simulink model "ex2_4"  (Simulink 7.8)
settings: Solver=ode45  StartTime=0.0  StopTime=1000.0  MaxStep=1  MinStep=1e-3  RelTol=1e-3
libraries: simulink x2
settings Model: Creator=Luke  LastModifiedBy=Luke

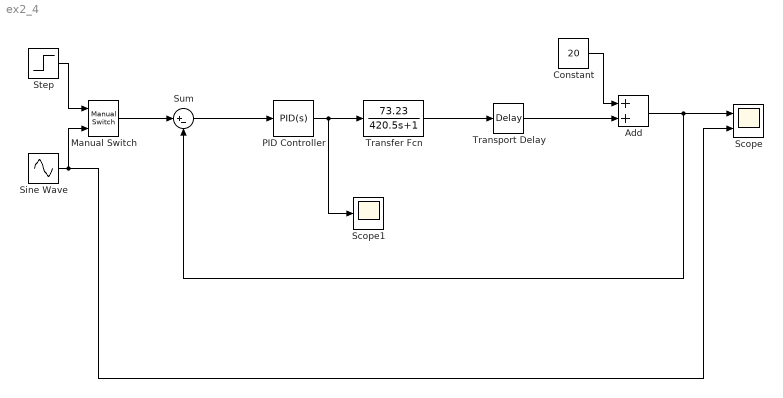
== system ex2_4 ==
  Add : Sum
  Constant : Constant  Value=20
  Manual Switch : simulink/Signal Routing/Manual Switch  sw=1  action=0  varsize=off
  PID Controller : simulink/Continuous/PID Controller  Controller=PID  TimeDomain=Continuous-time  SampleTime=1  IntegratorMethod=Forward Euler  FilterMethod=Forward Euler  Form=Parallel  P=0.6*0.2  I=(1.2*0.2)/110  D=(3*0.2*110)/40  N=15  InitialConditionSource=internal  InitialConditionForIntegrator=0  InitialConditionForFilter=0  ExternalReset=none  LimitOutput=off  UpperSaturationLimit=inf  LowerSaturationLimit=-inf  LinearizeAsGain=off  AntiWindupMode=none  Kb=1  TrackingMode=off  Kt=1  PParamMin=[]  PParamMax=[]  IParamMin=[]  IParamMax=[]  DParamMin=[]  DParamMax=[]  NParamMin=[]  NParamMax=[]  KbParamMin=[]  KbParamMax=[]  KtParamMin=[]  KtParamMax=[]  POutMin=[]  POutMax=[]  IOutMin=[]  IOutMax=[]  DOutMin=[]  DOutMax=[]  NOutMin=[]  NOutMax=[]  KbOutMin=[]  KbOutMax=[]  KtOutMin=[]  KtOutMax=[]  IntegratorOutMin=[]  IntegratorOutMax=[]  FilterOutMin=[]  FilterOutMax=[]  SumOutMin=[]  SumOutMax=[]  SumI1OutMin=[]  SumI1OutMax=[]  SumI2OutMin=[]  SumI2OutMax=[]  SumI3OutMin=[]  SumI3OutMax=[]  SumDOutMin=[]  SumDOutMax=[]  SaturationOutMin=[]  SaturationOutMax=[]  IntegratorContinuousStateAttributes=''  IntegratorStateMustResolveToSignalObject=off  IntegratorRTWStateStorageClass=Auto  FilterContinuousStateAttributes=''  FilterStateMustResolveToSignalObject=off  FilterRTWStateStorageClass=Auto
  Scope : Scope  NumInputPorts=2
      settings: YMin=20~-5  YMax=21.75~5
  Scope1 : Scope
      settings: YMin=20  YMax=21.75
  Sine Wave : Sin  Amplitude=2  Bias=20  Frequency=0.005  SampleTime=0
  Step : Step  Before=20  After=21  SampleTime=0
  Sum : Sum  Inputs=|+-
  Transfer Fcn : TransferFcn  Numerator=[73.23]  Denominator=[420.5 1]
  Transport Delay : TransportDelay  DelayTime=30  BufferSize=16635
  wires:
  Constant/1 -> Add/1
  Transfer Fcn/1 -> Transport Delay/1
  Transport Delay/1 -> Add/2
  Add/1 -> Sum/2, Scope/1
  Sum/1 -> PID Controller/1
  PID Controller/1 -> Transfer Fcn/1, Scope1/1
  Manual Switch/1 -> Sum/1
  Step/1 -> Manual Switch/1
  Sine Wave/1 -> Manual Switch/2, Scope/2
